simulink model "modele_bf"  (R2026a)
settings: Solver=VariableStepAuto  StopTime=40
undefined symbols (not defined in the file or in its folder): Aobs, Bobs, Cobs, d1_nom, d2, Dobs, K, k, Ki, km, Kr, ky, m1, m2
settings Model: Creator=flo  LastModifiedBy=floberg

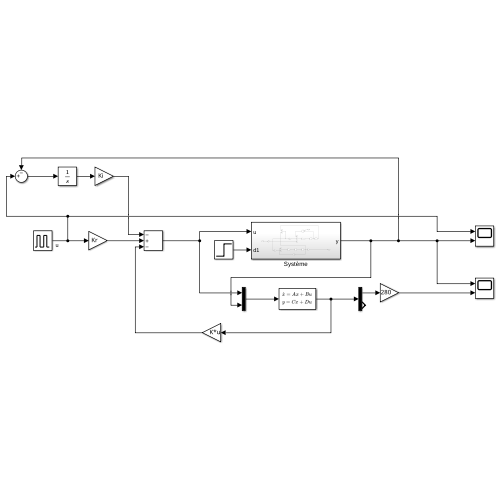
[thumbnail: Simulink's stored preview of the top-level diagram]
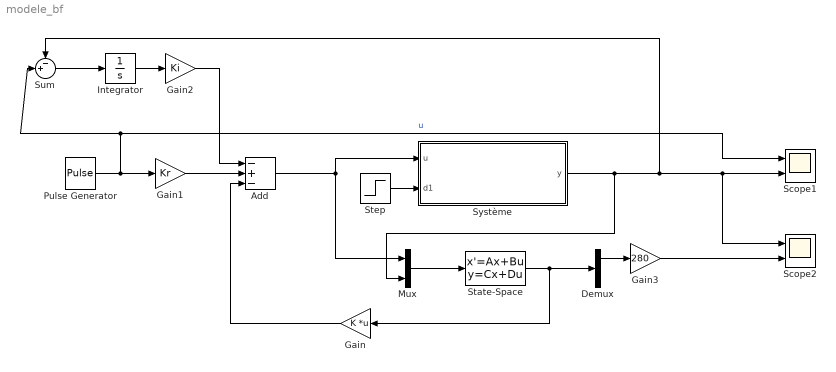
== system modele_bf ==
  Add : Sum  Inputs=-+-
  Demux : Demux  Outputs=[1,3]
  Gain : Gain  Gain=K  Multiplication=Matrix(K*u)
  Gain1 : Gain  Gain=Kr
  Gain2 : Gain  Gain=Ki
  Gain3 : Gain  Gain=280
  Integrator : Integrator
  Mux : Mux  Inputs=2
  Pulse Generator : DiscretePulseGenerator  PulseType=Time based  Period=3  PulseWidth=50
  Scope1 : Scope  NumInputPorts=2
      settings: ActiveDisplayYMinimum=-0.16140328672463361  ActiveDisplayYMaximum=1.1613880429831567
  Scope2 : Scope  NumInputPorts=2
      settings: ActiveDisplayYMinimum=-0.16140328672463361  ActiveDisplayYMaximum=1.1613880429831567
  State-Space : StateSpace  A=Aobs  B=Bobs  C=Cobs  D=Dobs  InitialCondition=0
  Step : Step  Time=20  InitialValue=d1_nom  FinalValue=d1_nom*2  SampleTime=0
  Sum : Sum  Inputs=-+|
  Système : Subsystem
  wires:
  Système/1(y) -> Mux/2, Scope2/1, Scope1/2, Sum/1
  State-Space/1 -> Gain/1, Demux/1
  Pulse Generator/1 -> Scope1/1, Sum/2, Gain1/1  "u"
  Sum/1 -> Integrator/1
  Gain1/1 -> Add/2
  Integrator/1 -> Gain2/1
  Gain2/1 -> Add/1
  Gain/1 -> Add/3
  Add/1 -> Mux/1, Système/1(u)
  Mux/1 -> State-Space/1
  Step/1 -> Système/2(d1)
  Demux/1 -> Gain3/1
  Gain3/1 -> Scope2/2

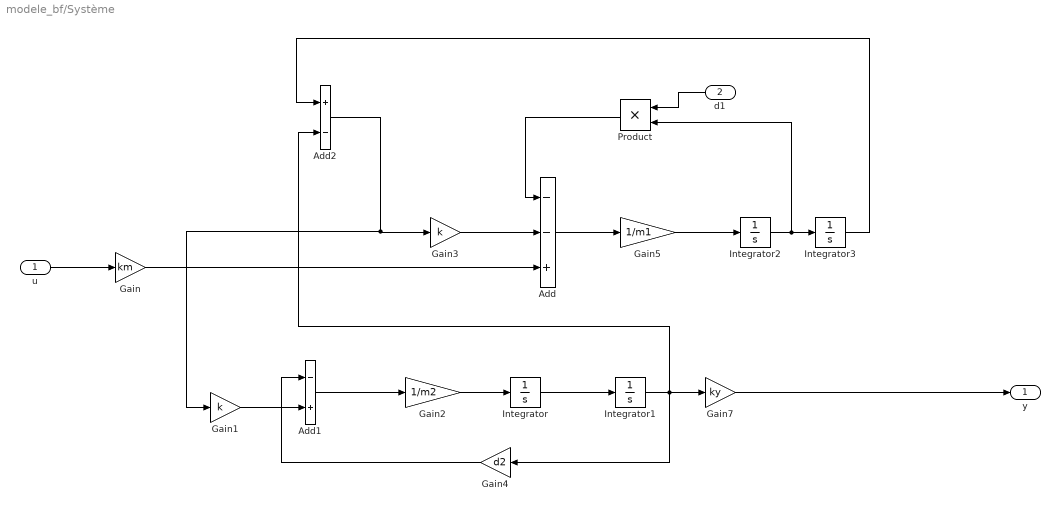
== system modele_bf/Système ==
  u : Inport
  d1 : Inport  Port=2
  Add : Sum  Inputs=--+
  Add1 : Sum  Inputs=-+
  Add2 : Sum  Inputs=+-
  Gain : Gain  Gain=km
  Gain1 : Gain  Gain=k
  Gain2 : Gain  Gain=1/m2
  Gain3 : Gain  Gain=k
  Gain4 : Gain  Gain=d2
  Gain5 : Gain  Gain=1/m1
  Gain7 : Gain  Gain=ky
  Integrator{,1..3} (4 alike) : Integrator
  Product : Product
  y : Outport
  wires:
  Integrator3/1 -> Add2/1
  Add2/1 -> Gain1/1, Gain3/1
  Integrator2/1 -> Product/2, Integrator3/1
  Gain2/1 -> Integrator/1
  Integrator/1 -> Integrator1/1
  Gain3/1 -> Add/2
  Add1/1 -> Gain2/1
  Gain1/1 -> Add1/2
  Gain4/1 -> Add1/1
  Product/1 -> Add/1
  Gain5/1 -> Integrator2/1
  u/1 -> Gain/1
  Add/1 -> Gain5/1
  Gain/1 -> Add/3
  Integrator1/1 -> Gain7/1, Gain4/1, Add2/2
  Gain7/1 -> y/1
  d1/1 -> Product/1
